simulink model "Time_example"  (R2015a)
settings: Solver=ode1  SolverMode=SingleTasking  StartTime=0.0  StopTime=Inf  FixedStep=0.0001  RelTol=1e-3
PostLoadFcn:
  | , if any(exist('dsrtsu_mdlpostloadfcn', 'file') == [2, 3, 6]), try dsrtsu_mdlpostloadfcn('Execute', bdroot); catch fprintf('Error in PostLoadFcn (dsrtsu_mdlpostloadfcn) for model "%s":\n %s\n', bdroot, lasterr); end, end,
libraries: rti1401lib_I_base x12, rtilib1401 x1
settings Model: RTICANMMDATA=struct('GeneralSetupData',struct('modelroot','E:\Support\RTI.2016.05.17.008','generalsettings',struct('filesettings',struct('destfolder',struct('Name','RTICANMM_FILES','Check',1),'buildfolder',struct('Name','.','Check',1),'AbsDestfolder',struct('Name','E:\Support\RTI.2016.05.17.008\RTICANMM_FILES'),'AbsBuildfolder',struct('Name','E:\Support\RTI.2016.05.17.008'))),'options',struct('addpaths',1,'rmpaths',1,'addtrcexclusion',logical(1),'cannavigator',struct('checkmonitoring',0),'show_usrtrc',0,'use_usrtrc',0),'advanced',struct('options',[1 1 1 1 1 1 1 1 1 1 1 1 1 1 1 1 1 1 1 1 1 1 1 1 1 1 1 1 1 1 1 1 1 1 1 1 1 1 1 1 1 1 1 1 1 1 1 1 1 1 1 1 1 1 1 1 1 1 1 1 1 1 1 1 1 1 1 1 1 1 1 1 1 1 1 1 1 1 1 1 1 1 1 1 1 1 1 1 1 1 1 1 1 1 1 1 1 1 1 1]),'MPSetup',{{}},'modelname','smd_1401_sl','block','smd_1401_sl'))  RTILINMMDATA=struct('GeneralSetupData',[])  DSRTSU_INTERNAL_RTI_VER=470  DSRTSU_INTERNAL_RTI_TYPE=rti1401  DSRTSU_INTERNAL_RTIFLEXRAYCONFIG=80  DSRTSU_INTERNAL_RTIFPGA=60  DSAPPLBUILDDATA=struct('workDir','E:\Support\RTI.2016.05.17.008','mpMainModel','smd_1401_sl','modelName','smd_1401_sl','isRTIMp',logical(0),'VerboseLevel',0,'modelHandle',3.000244140625,'mpMainHandle',3.000244140625,'buildDir','.\smd_1401_sl_rti1401','IsCodeGen',logical(1))  CovSFcnEnable=off  ExtModeTrigMode=oneshot  ExtModeArmWhenConnect=off  ExtModeAutoUpdateStatusClock=off  Creator=dSPACE GmbH  LastModifiedBy=Powertrain_software
settings DataIOCC: SignalLoggingSaveFormat=ModelDataLogs
settings OptimizationCC: BlockReduction=off  ConditionallyExecuteInputs=off  OptimizeBlockIOStorage=off  BufferReuse=off  GlobalBufferReuse=off  ExpressionFolding=off  ExpressionDepthLimit=2147483647  LocalBlockOutputs=off  InitFltsAndDblsToZero=on
settings DebuggingCC: SaveWithParameterizedLinksMsg=none  UnderspecifiedInitializationDetection=Classic  MergeDetectMultiDrivingBlocksExec=none  SignalResolutionControl=TryResolveAllWithWarning  SolverPrmCheckMsg=warning  MultiTaskDSMMsg=warning  MultiTaskCondExecSysMsg=none  MultiTaskRateTransMsg=warning  TasksWithSamePriorityMsg=none  FcnCallInpInsideContextMsg=UseLocalSettings  StateNameClashWarn=warning
settings HardwareCC: ProdLargestAtomicInteger=Integer  ProdLargestAtomicFloat=Float  ProdIntDivRoundTo=Zero  ProdEndianess=BigEndian  ProdHWDeviceType=Generic->Custom  TargetIntDivRoundTo=Zero  TargetEndianess=BigEndian  TargetHWDeviceType=Generic->Custom
settings RTWCC: SystemTargetFile=rti1401.tlc  MakeCommand=make_rti  TemplateMakefile=rti1401.tmf  Description=dSPACE DS1401 Hardware Platform  RTWVerbose=off
settings STFCustomTargetCC: TargetFcnLib=ansi_tfl_tmw.mat  GenerateSampleERTMain=off  ParMdlRefBuildCompliant=on  GeneratePreprocessorConditionals=Disable all  ERTCustomFileBanners=off  SupportNonInlinedSFcns=on  SupportVariableSizeSignals=off  MATLABClassNameForMDSCustomization=Simulink.SoftwareTarget.GRTCustomization  GRTInterface=on  SystemTargetFile=rti1401.tlc
settings GRTTargetCC: TargetFcnLib=ansi_tfl_tmw.mat  CompOptLevelCompliant=off  ConcurrentExecutionCompliant=off  CombineOutputUpdateFcns=off  MatFileLogging=off  CPPClassGenCompliant=off  GRTInterface=on  ExtModeMexFile=noextcomm

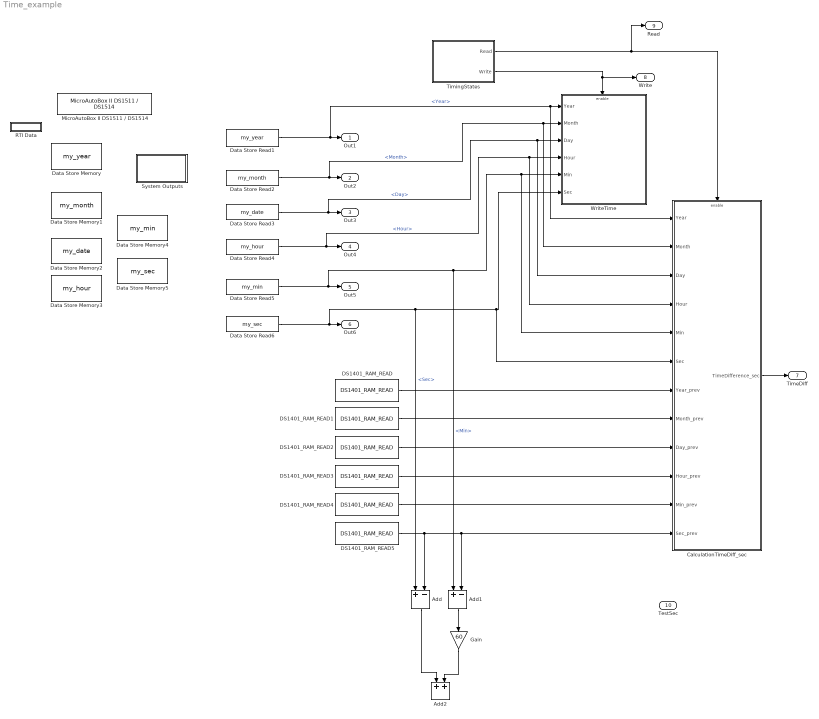
== system Time_example ==
  Add : Sum  Inputs=+-
  Add1 : Sum  Inputs=+-
  Add2 : Sum
  CalculationTimeDiff_sec : Subsystem  TreatAsAtomicUnit=on
  DS1401_RAM_READ : rti1401lib_I_base/DS1401_RAM_READ  DataType=Int8  Address=0  SampleTime=-1  Reserved1=[]  Reserved2=[]  Reserved3=[]  Reserved4=[]  DSProperties=struct('RTI',struct('Version',uint32(1),'BlockType',struct('isSLSource',uint8(1),'isSLSink',uint8(0),'isHWSource',uint8(0),'isHWSink',uint8(1),'isSetup',uint8(0),'isInline',uint8(1),'isNonInline',uint8(1),'isInterrupt',uint8(0),'isChannelwise',uint8(0)),'IOBoardType',{{'DS1401','BASE'}},'UnitType','RAM','Identifier','RAMREAD','DialogType','SL','BlockSet','NONE','SlaveProcessor','NONE'))  RTIBlockInterface=struct('OutputPortsActive',1,'BlockDisplay',{{['From\nnon-volatile RAM'],'center'}},'IconTransparency','off','InitLevel',1,'BlockName',struct('Token',{{'DS1401_RAM_READ'}}),'MaskDescription',['Provide read access from non-volatile Real-Time-Clock user RAM.'])  RTIBlockParameters=struct('DataType',{{1,'ON',[1 8]}},'Address',{{0,'ON','DataType',[0 1 2 3 4 5 6 7 8 9 10 11 12 13 14 15;0 1 2 3 4 5 6 7 8 9 10 11 12 13 14 15;0 0 2 2 4 4 6 6 8 8 10 10 12 12 14 14;0 0 2 2 4 4 6 6 8 8 10 10 12 12 14 14;0 0 0 0 4 4 4 4 8 8 8 8 12 12 12 12;0 0 0 0 4 4 4 4 8 8 8 8 12 12 12 12;0 0 0 0 4 4 4 4 8 8 8 8 12 12 12 12;0 0 0 0 0 0 0 0 8 8 8 8 8 8 8 8]}},'SampleTime',{{-1,'OFF',[]}})  RTISFcnParameters=struct('DataType','double','Address','double','SampleTime','double')  RTIBlockParaDefault=struct('DataType',8,'Address',0,'SampleTime',-1)
  DS1401_RAM_READ1 : rti1401lib_I_base/DS1401_RAM_READ  DataType=Int8  Address=1  SampleTime=-1  Reserved1=[]  Reserved2=[]  Reserved3=[]  Reserved4=[]  DSProperties=struct('RTI',struct('Version',uint32(1),'BlockType',struct('isSLSource',uint8(1),'isSLSink',uint8(0),'isHWSource',uint8(0),'isHWSink',uint8(1),'isSetup',uint8(0),'isInline',uint8(1),'isNonInline',uint8(1),'isInterrupt',uint8(0),'isChannelwise',uint8(0)),'IOBoardType',{{'DS1401','BASE'}},'UnitType','RAM','Identifier','RAMREAD','DialogType','SL','BlockSet','NONE','SlaveProcessor','NONE'))  RTIBlockInterface=struct('OutputPortsActive',1,'BlockDisplay',{{['From\nnon-volatile RAM'],'center'}},'IconTransparency','off','InitLevel',1,'BlockName',struct('Token',{{'DS1401_RAM_READ'}}),'MaskDescription',['Provide read access from non-volatile Real-Time-Clock user RAM.'])  RTIBlockParameters=struct('DataType',{{1,'ON',[1 8]}},'Address',{{1,'ON','DataType',[0 1 2 3 4 5 6 7 8 9 10 11 12 13 14 15;0 1 2 3 4 5 6 7 8 9 10 11 12 13 14 15;0 0 2 2 4 4 6 6 8 8 10 10 12 12 14 14;0 0 2 2 4 4 6 6 8 8 10 10 12 12 14 14;0 0 0 0 4 4 4 4 8 8 8 8 12 12 12 12;0 0 0 0 4 4 4 4 8 8 8 8 12 12 12 12;0 0 0 0 4 4 4 4 8 8 8 8 12 12 12 12;0 0 0 0 0 0 0 0 8 8 8 8 8 8 8 8]}},'SampleTime',{{-1,'OFF',[]}})  RTISFcnParameters=struct('DataType','double','Address','double','SampleTime','double')  RTIBlockParaDefault=struct('DataType',8,'Address',0,'SampleTime',-1)
  DS1401_RAM_READ2 : rti1401lib_I_base/DS1401_RAM_READ  DataType=Int8  Address=2  SampleTime=-1  Reserved1=[]  Reserved2=[]  Reserved3=[]  Reserved4=[]  DSProperties=struct('RTI',struct('Version',uint32(1),'BlockType',struct('isSLSource',uint8(1),'isSLSink',uint8(0),'isHWSource',uint8(0),'isHWSink',uint8(1),'isSetup',uint8(0),'isInline',uint8(1),'isNonInline',uint8(1),'isInterrupt',uint8(0),'isChannelwise',uint8(0)),'IOBoardType',{{'DS1401','BASE'}},'UnitType','RAM','Identifier','RAMREAD','DialogType','SL','BlockSet','NONE','SlaveProcessor','NONE'))  RTIBlockInterface=struct('OutputPortsActive',1,'BlockDisplay',{{['From\nnon-volatile RAM'],'center'}},'IconTransparency','off','InitLevel',1,'BlockName',struct('Token',{{'DS1401_RAM_READ'}}),'MaskDescription',['Provide read access from non-volatile Real-Time-Clock user RAM.'])  RTIBlockParameters=struct('DataType',{{1,'ON',[1 8]}},'Address',{{2,'ON','DataType',[0 1 2 3 4 5 6 7 8 9 10 11 12 13 14 15;0 1 2 3 4 5 6 7 8 9 10 11 12 13 14 15;0 0 2 2 4 4 6 6 8 8 10 10 12 12 14 14;0 0 2 2 4 4 6 6 8 8 10 10 12 12 14 14;0 0 0 0 4 4 4 4 8 8 8 8 12 12 12 12;0 0 0 0 4 4 4 4 8 8 8 8 12 12 12 12;0 0 0 0 4 4 4 4 8 8 8 8 12 12 12 12;0 0 0 0 0 0 0 0 8 8 8 8 8 8 8 8]}},'SampleTime',{{-1,'OFF',[]}})  RTISFcnParameters=struct('DataType','double','Address','double','SampleTime','double')  RTIBlockParaDefault=struct('DataType',8,'Address',0,'SampleTime',-1)
  DS1401_RAM_READ3 : rti1401lib_I_base/DS1401_RAM_READ  DataType=Int8  Address=3  SampleTime=-1  Reserved1=[]  Reserved2=[]  Reserved3=[]  Reserved4=[]  DSProperties=struct('RTI',struct('Version',uint32(1),'BlockType',struct('isSLSource',uint8(1),'isSLSink',uint8(0),'isHWSource',uint8(0),'isHWSink',uint8(1),'isSetup',uint8(0),'isInline',uint8(1),'isNonInline',uint8(1),'isInterrupt',uint8(0),'isChannelwise',uint8(0)),'IOBoardType',{{'DS1401','BASE'}},'UnitType','RAM','Identifier','RAMREAD','DialogType','SL','BlockSet','NONE','SlaveProcessor','NONE'))  RTIBlockInterface=struct('OutputPortsActive',1,'BlockDisplay',{{['From\nnon-volatile RAM'],'center'}},'IconTransparency','off','InitLevel',1,'BlockName',struct('Token',{{'DS1401_RAM_READ'}}),'MaskDescription',['Provide read access from non-volatile Real-Time-Clock user RAM.'])  RTIBlockParameters=struct('DataType',{{1,'ON',[1 8]}},'Address',{{3,'ON','DataType',[0 1 2 3 4 5 6 7 8 9 10 11 12 13 14 15;0 1 2 3 4 5 6 7 8 9 10 11 12 13 14 15;0 0 2 2 4 4 6 6 8 8 10 10 12 12 14 14;0 0 2 2 4 4 6 6 8 8 10 10 12 12 14 14;0 0 0 0 4 4 4 4 8 8 8 8 12 12 12 12;0 0 0 0 4 4 4 4 8 8 8 8 12 12 12 12;0 0 0 0 4 4 4 4 8 8 8 8 12 12 12 12;0 0 0 0 0 0 0 0 8 8 8 8 8 8 8 8]}},'SampleTime',{{-1,'OFF',[]}})  RTISFcnParameters=struct('DataType','double','Address','double','SampleTime','double')  RTIBlockParaDefault=struct('DataType',8,'Address',0,'SampleTime',-1)
  DS1401_RAM_READ4 : rti1401lib_I_base/DS1401_RAM_READ  DataType=Int8  Address=4  SampleTime=-1  Reserved1=[]  Reserved2=[]  Reserved3=[]  Reserved4=[]  DSProperties=struct('RTI',struct('Version',uint32(1),'BlockType',struct('isSLSource',uint8(1),'isSLSink',uint8(0),'isHWSource',uint8(0),'isHWSink',uint8(1),'isSetup',uint8(0),'isInline',uint8(1),'isNonInline',uint8(1),'isInterrupt',uint8(0),'isChannelwise',uint8(0)),'IOBoardType',{{'DS1401','BASE'}},'UnitType','RAM','Identifier','RAMREAD','DialogType','SL','BlockSet','NONE','SlaveProcessor','NONE'))  RTIBlockInterface=struct('OutputPortsActive',1,'BlockDisplay',{{['From\nnon-volatile RAM'],'center'}},'IconTransparency','off','InitLevel',1,'BlockName',struct('Token',{{'DS1401_RAM_READ'}}),'MaskDescription',['Provide read access from non-volatile Real-Time-Clock user RAM.'])  RTIBlockParameters=struct('DataType',{{1,'ON',[1 8]}},'Address',{{4,'ON','DataType',[0 1 2 3 4 5 6 7 8 9 10 11 12 13 14 15;0 1 2 3 4 5 6 7 8 9 10 11 12 13 14 15;0 0 2 2 4 4 6 6 8 8 10 10 12 12 14 14;0 0 2 2 4 4 6 6 8 8 10 10 12 12 14 14;0 0 0 0 4 4 4 4 8 8 8 8 12 12 12 12;0 0 0 0 4 4 4 4 8 8 8 8 12 12 12 12;0 0 0 0 4 4 4 4 8 8 8 8 12 12 12 12;0 0 0 0 0 0 0 0 8 8 8 8 8 8 8 8]}},'SampleTime',{{-1,'OFF',[]}})  RTISFcnParameters=struct('DataType','double','Address','double','SampleTime','double')  RTIBlockParaDefault=struct('DataType',8,'Address',0,'SampleTime',-1)
  DS1401_RAM_READ5 : rti1401lib_I_base/DS1401_RAM_READ  DataType=Int8  Address=5  SampleTime=-1  Reserved1=[]  Reserved2=[]  Reserved3=[]  Reserved4=[]  DSProperties=struct('RTI',struct('Version',uint32(1),'BlockType',struct('isSLSource',uint8(1),'isSLSink',uint8(0),'isHWSource',uint8(0),'isHWSink',uint8(1),'isSetup',uint8(0),'isInline',uint8(1),'isNonInline',uint8(1),'isInterrupt',uint8(0),'isChannelwise',uint8(0)),'IOBoardType',{{'DS1401','BASE'}},'UnitType','RAM','Identifier','RAMREAD','DialogType','SL','BlockSet','NONE','SlaveProcessor','NONE'))  RTIBlockInterface=struct('OutputPortsActive',1,'BlockDisplay',{{['From\nnon-volatile RAM'],'center'}},'IconTransparency','off','InitLevel',1,'BlockName',struct('Token',{{'DS1401_RAM_READ'}}),'MaskDescription',['Provide read access from non-volatile Real-Time-Clock user RAM.'])  RTIBlockParameters=struct('DataType',{{1,'ON',[1 8]}},'Address',{{5,'ON','DataType',[0 1 2 3 4 5 6 7 8 9 10 11 12 13 14 15;0 1 2 3 4 5 6 7 8 9 10 11 12 13 14 15;0 0 2 2 4 4 6 6 8 8 10 10 12 12 14 14;0 0 2 2 4 4 6 6 8 8 10 10 12 12 14 14;0 0 0 0 4 4 4 4 8 8 8 8 12 12 12 12;0 0 0 0 4 4 4 4 8 8 8 8 12 12 12 12;0 0 0 0 4 4 4 4 8 8 8 8 12 12 12 12;0 0 0 0 0 0 0 0 8 8 8 8 8 8 8 8]}},'SampleTime',{{-1,'OFF',[]}})  RTISFcnParameters=struct('DataType','double','Address','double','SampleTime','double')  RTIBlockParaDefault=struct('DataType',8,'Address',0,'SampleTime',-1)
  Data Store Memory : DataStoreMemory  DataStoreName=my_year  ReadBeforeWriteMsg=warning  WriteAfterWriteMsg=warning  WriteAfterReadMsg=warning
      settings: RTWStateStorageClass=ExportedGlobal
  Data Store Memory1 : DataStoreMemory  DataStoreName=my_month  ReadBeforeWriteMsg=warning  WriteAfterWriteMsg=warning  WriteAfterReadMsg=warning
      settings: RTWStateStorageClass=ExportedGlobal
  Data Store Memory2 : DataStoreMemory  DataStoreName=my_date  ReadBeforeWriteMsg=warning  WriteAfterWriteMsg=warning  WriteAfterReadMsg=warning
      settings: RTWStateStorageClass=ExportedGlobal
  Data Store Memory3 : DataStoreMemory  DataStoreName=my_hour  ReadBeforeWriteMsg=warning  WriteAfterWriteMsg=warning  WriteAfterReadMsg=warning
      settings: RTWStateStorageClass=ExportedGlobal
  Data Store Memory4 : DataStoreMemory  DataStoreName=my_min  ReadBeforeWriteMsg=warning  WriteAfterWriteMsg=warning  WriteAfterReadMsg=warning
      settings: RTWStateStorageClass=ExportedGlobal
  Data Store Memory5 : DataStoreMemory  DataStoreName=my_sec  ReadBeforeWriteMsg=warning  WriteAfterWriteMsg=warning  WriteAfterReadMsg=warning
      settings: RTWStateStorageClass=ExportedGlobal
  Data Store Read1 : DataStoreRead  DataStoreName=my_year
  Data Store Read2 : DataStoreRead  DataStoreName=my_month
  Data Store Read3 : DataStoreRead  DataStoreName=my_date
  Data Store Read4 : DataStoreRead  DataStoreName=my_hour
  Data Store Read5 : DataStoreRead  DataStoreName=my_min
  Data Store Read6 : DataStoreRead  DataStoreName=my_sec
  Gain : Gain  Gain=60
  MicroAutoBox II DS1511 / DS1514 : rtilib1401/MicroAutoBox II DS1511 // DS1514  SystemSampleTime=-1
  RTI Data : Subsystem  Tag=struct('RTIDataServer',struct('RTIDataServerVs','2','RTIModelDescription','struct(''main'',''Time_example'',''sub'','''',''isMp'',0)'))  LoadFcn="if exist('rtidc'), try,  rtidc('DataHostBlockClbLoad', gcbh); catch, disp(['Warning: ''LoadFcn'' for RTI Data block failed: ' lasterr]); end, end,"  mask(RTI_DATA_HOST){}
      mask help:
      | RTI Data Block.
      | This block is used by RTI to store internal model-dependent data.
      | Please keep this block on the root level of the model. Deleting this block will result in data loss.
      |
      | NEVER DELETE OR COPY THIS BLOCK!
      settings: CopyFcn="if exist('rtidc'), try,  rtidc('DataHostBlockClbCopy', gcbh); catch, disp(['Warning: ''CopyFcn'' for RTI Data block failed: ' lasterr]); end, end,"  DeleteFcn="if exist('rtidc'), try,  rtidc('DataHostBlockClbDelete', gcbh); catch, disp(['Warning: ''DeleteFcn'' for RTI Data block failed: ' lasterr]); end, end,"  ModelCloseFcn="if exist('rtidc'), try,  rtidc('DataHostBlockClbModelClose', gcbh); catch, disp(['Warning: ''ModelCloseFcn'' for RTI Data block failed: ' lasterr]); end, end,"  PreSaveFcn="if exist('rtidc'), try,  rtidc('DataHostBlockClbPreSave', gcbh); catch, disp(['Warning: ''PreSaveFcn'' for RTI Data block failed: ' lasterr]); end, end,"  PostSaveFcn="if exist('rtidc'), try,  rtidc('DataHostBlockClbPostSave', gcbh); catch, disp(['Warning: ''PostSaveFcn'' for RTI Data block failed: ' lasterr]); end, end,"  NameChangeFcn="if exist('rtidc'), try,  rtidc('DataHostBlockClbNameChange', gcbh); catch, disp(['Warning: ''NameChangeFcn'' for RTI Data block failed: ' lasterr]); end, end,"
      mask Help:
      | RTI Data Block.
      | This block is used by RTI to store internal model-dependent data.
      | Please keep this block on the root level of the model. Deleting this block will result in data loss.
      | 
      | NEVER DELETE OR COPY THIS BLOCK!
      mask Display:
      | text(0.5, 0.5, 'RTI Data', 'HorizontalAlignment', 'center');
      | plot([1 0]);
  System Outputs : Subsystem  mask(System Outputs){ShowInLibBrowser=0}
      mask prompts: ShowInLibBrowser "Simulink:masks:CustCodeMaskParam1_MP"
      settings: CopyFcn=cccopyfcn(gcb)  OpenFcn=ccopenfcn('System Outputs Function')
      mask Help: eval('feval(''rtwprivate'',''rtwhelpview'',''rtw_sys_outputs_block'')');
      mask Display: disp('System\nOutputs');
  TimingStates : Stateflow chart  TreatAsAtomicUnit=on
  WriteTime : Subsystem  TreatAsAtomicUnit=on
  Out1 : Outport
  Out2 : Outport  Port=2
  Out3 : Outport  Port=3
  Out4 : Outport  Port=4
  Out5 : Outport  Port=5
  Out6 : Outport  Port=6
  TimeDiff : Outport  Port=7
  Write : Outport  Port=8
  Read : Outport  Port=9
  TestSec : Outport  Port=10
  wires:
  TimingStates/1(Read) -> Read/1, CalculationTimeDiff_sec/Enable
  TimingStates/2(Write) -> Write/1, WriteTime/Enable
  Data Store Read1/1 -> CalculationTimeDiff_sec/1(Year), WriteTime/1(Year), Out1/1  "<Year>"
  Data Store Read5/1 -> Add1/1, CalculationTimeDiff_sec/5(Min), WriteTime/5(Min), Out5/1  "<Min>"
  Data Store Read4/1 -> CalculationTimeDiff_sec/4(Hour), WriteTime/4(Hour), Out4/1  "<Hour>"
  Data Store Read2/1 -> CalculationTimeDiff_sec/2(Month), WriteTime/2(Month), Out2/1  "<Month>"
  Data Store Read6/1 -> CalculationTimeDiff_sec/6(Sec), WriteTime/6(Sec), Add/1, Out6/1  "<Sec>"
  Data Store Read3/1 -> CalculationTimeDiff_sec/3(Day), WriteTime/3(Day), Out3/1  "<Day>"
  CalculationTimeDiff_sec/1(TimeDifference_sec) -> TimeDiff/1
  DS1401_RAM_READ5/1 -> CalculationTimeDiff_sec/12(Sec_prev), Add1/2, Add/2
  DS1401_RAM_READ4/1 -> CalculationTimeDiff_sec/11(Min_prev)
  DS1401_RAM_READ3/1 -> CalculationTimeDiff_sec/10(Hour_prev)
  DS1401_RAM_READ2/1 -> CalculationTimeDiff_sec/9(Day_prev)
  DS1401_RAM_READ1/1 -> CalculationTimeDiff_sec/8(Month_prev)
  DS1401_RAM_READ/1 -> CalculationTimeDiff_sec/7(Year_prev)
  Add1/1 -> Gain/1
  Add/1 -> Add2/1
  Gain/1 -> Add2/2

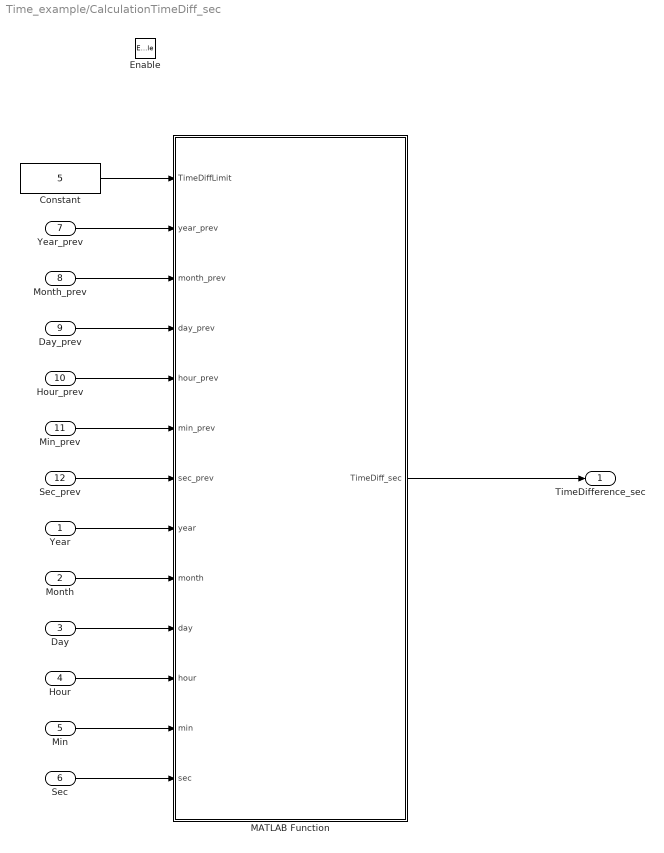
== system Time_example/CalculationTimeDiff_sec ==
  Year : Inport
  Month : Inport  Port=2
  Day : Inport  Port=3
  Hour : Inport  Port=4
  Min : Inport  Port=5
  Sec : Inport  Port=6
  Year_prev : Inport  Port=7
  Month_prev : Inport  Port=8
  Day_prev : Inport  Port=9
  Hour_prev : Inport  Port=10
  Min_prev : Inport  Port=11
  Sec_prev : Inport  Port=12
  Enable : EnablePort
  Constant : Constant  Value=5  OutDataTypeStr=int8
  MATLAB Function : MATLAB Function  TreatAsAtomicUnit=on
  TimeDifference_sec : Outport
  wires:
  MATLAB Function/1(TimeDiff_sec) -> TimeDifference_sec/1
  Constant/1 -> MATLAB Function/1(TimeDiffLimit)
  Sec_prev/1 -> MATLAB Function/7(sec_prev)
  Year/1 -> MATLAB Function/8(year)
  Month/1 -> MATLAB Function/9(month)
  Day/1 -> MATLAB Function/10(day)
  Hour/1 -> MATLAB Function/11(hour)
  Min/1 -> MATLAB Function/12(min)
  Sec/1 -> MATLAB Function/13(sec)
  Min_prev/1 -> MATLAB Function/6(min_prev)
  Day_prev/1 -> MATLAB Function/4(day_prev)
  Hour_prev/1 -> MATLAB Function/5(hour_prev)
  Month_prev/1 -> MATLAB Function/3(month_prev)
  Year_prev/1 -> MATLAB Function/2(year_prev)

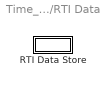
== system Time_example/RTI Data ==
  RTI Data Store : Subsystem  Tag="struct('private',struct('version',struct('dsVer',uint32(2),'dsVerCreation',uint32(2),'RTI',struct('ver','7.5p2','type','RTI1401')),'access',struct('type','Model','isPerm',1,'created',['19-May-2016 14:11:30'],'modified',['20-May-2016 18:16:36'],'location','')),'public',struct('main',struct('data',[]),'sub',struct('name',{{'Time_example'}},'data',{{struct('TH',struct('thTaskInfo',struct('taskType',{'TIMER','HWINT','TMRINT','SWINT','GLINT'},'tasksNumOf',{1,0,0,0,0},'srcIds',{{'TIMERA'},{},{},{},{}},'taskNames',{{['Timer Task 1']},{},{},{},{}})),'th_tc',struct('dataType','TASK','taskGroupId','','taskGroupList',{{}},'taskSchedulingPolicy','FCFS','taskType','TIMER','blkh',-1,'srcId','TIMERA','srcSgnName',['Timer A interrupt'],'srcCpuName','','taskName',['Timer Task 1  [0.0001] s'],'taskNameDisplayExt','','smplTime',0.0001,'smplTimeOffs',0,'hasFixedPriority',0,'priority',1,'hasFixedOvc',0,'ovcType',1,'ovcMax',1),'tc_th',struct('dataType','TASK','taskGroupId','','taskGroupList',{{}},'taskSchedulingPolicy','FCFS','taskType','TIMER','blkh',-1,'srcId','TIMERA','srcSgnName',['Timer A interrupt'],'srcCpuName','','taskName',['Timer Task 1  [0.0001] s'],'taskNameDisplayExt','','smplTime',0.0001,'smplTimeOffs',0,'hasFixedPriority',0,'priority',1,'hasFixedOvc',0,'ovcType',1,'ovcMax',1))}})))"  mask(RTI_DATA_STORE){}
      mask help:
      | RTI Data Store Block. This block is used by RTI to store internal model dependent data. Deleting this block will result in data loss.
      |
      | NEVER DELETE, COPY, OR MODIFY THIS BLOCK!
      mask Help:
      | RTI Data Store Block. This block is used by RTI to store internal model dependent data. Deleting this block will result in data loss.
      | 
      | NEVER DELETE, COPY, OR MODIFY THIS BLOCK!
      mask Display: text(0.5, 0.5, ' ', 'HorizontalAlignment', 'center');

== system Time_example/System Outputs ==

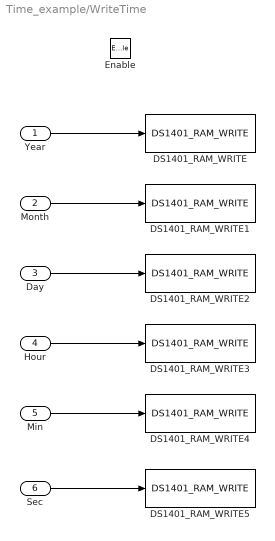
== system Time_example/WriteTime ==
  Year : Inport
  Month : Inport  Port=2
  Day : Inport  Port=3
  Hour : Inport  Port=4
  Min : Inport  Port=5
  Sec : Inport  Port=6
  Enable : EnablePort
  DS1401_RAM_WRITE : rti1401lib_I_base/DS1401_RAM_WRITE  DataType=Int8  Address=0  SampleTime=1  Reserved1=[]  Reserved2=[]  Reserved3=[]  Reserved4=[]  DSProperties=struct('RTI',struct('Version',uint32(1),'BlockType',struct('isSLSource',uint8(0),'isSLSink',uint8(1),'isHWSource',uint8(1),'isHWSink',uint8(1),'isSetup',uint8(0),'isInline',uint8(1),'isNonInline',uint8(1),'isInterrupt',uint8(0),'isChannelwise',uint8(0)),'IOBoardType',{{'DS1401','BASE'}},'UnitType','RAM','Identifier','RAMWRITE','DialogType','SL','BlockSet','NONE','SlaveProcessor','NONE'))  RTIBlockInterface=struct('InputPortsActive',1,'BlockDisplay',{{['To\nnon-volatile RAM'],'center'}},'IconTransparency','off','InitLevel',1,'BlockName',struct('Token',{{'DS1401_RAM_WRITE'}}),'MaskDescription',['Provide read access from non-volatile Real-Time-Clock user RAM.'])  RTIBlockParameters=struct('DataType',{{1,'ON',[1 8]}},'Address',{{0,'ON','DataType',[0 1 2 3 4 5 6 7 8 9 10 11 12 13 14 15;0 1 2 3 4 5 6 7 8 9 10 11 12 13 14 15;0 0 2 2 4 4 6 6 8 8 10 10 12 12 14 14;0 0 2 2 4 4 6 6 8 8 10 10 12 12 14 14;0 0 0 0 4 4 4 4 8 8 8 8 12 12 12 12;0 0 0 0 4 4 4 4 8 8 8 8 12 12 12 12;0 0 0 0 4 4 4 4 8 8 8 8 12 12 12 12;0 0 0 0 0 0 0 0 8 8 8 8 8 8 8 8]}},'SampleTime',{{1,'OFF',[]}})  RTISFcnParameters=struct('DataType','double','Address','double','SampleTime','double')  RTIBlockParaDefault=struct('DataType',8,'Address',0,'SampleTime',-1)
  DS1401_RAM_WRITE1 : rti1401lib_I_base/DS1401_RAM_WRITE  DataType=Int8  Address=1  SampleTime=1  Reserved1=[]  Reserved2=[]  Reserved3=[]  Reserved4=[]  DSProperties=struct('RTI',struct('Version',uint32(1),'BlockType',struct('isSLSource',uint8(0),'isSLSink',uint8(1),'isHWSource',uint8(1),'isHWSink',uint8(1),'isSetup',uint8(0),'isInline',uint8(1),'isNonInline',uint8(1),'isInterrupt',uint8(0),'isChannelwise',uint8(0)),'IOBoardType',{{'DS1401','BASE'}},'UnitType','RAM','Identifier','RAMWRITE','DialogType','SL','BlockSet','NONE','SlaveProcessor','NONE'))  RTIBlockInterface=struct('InputPortsActive',1,'BlockDisplay',{{['To\nnon-volatile RAM'],'center'}},'IconTransparency','off','InitLevel',1,'BlockName',struct('Token',{{'DS1401_RAM_WRITE'}}),'MaskDescription',['Provide read access from non-volatile Real-Time-Clock user RAM.'])  RTIBlockParameters=struct('DataType',{{1,'ON',[1 8]}},'Address',{{1,'ON','DataType',[0 1 2 3 4 5 6 7 8 9 10 11 12 13 14 15;0 1 2 3 4 5 6 7 8 9 10 11 12 13 14 15;0 0 2 2 4 4 6 6 8 8 10 10 12 12 14 14;0 0 2 2 4 4 6 6 8 8 10 10 12 12 14 14;0 0 0 0 4 4 4 4 8 8 8 8 12 12 12 12;0 0 0 0 4 4 4 4 8 8 8 8 12 12 12 12;0 0 0 0 4 4 4 4 8 8 8 8 12 12 12 12;0 0 0 0 0 0 0 0 8 8 8 8 8 8 8 8]}},'SampleTime',{{1,'OFF',[]}})  RTISFcnParameters=struct('DataType','double','Address','double','SampleTime','double')  RTIBlockParaDefault=struct('DataType',8,'Address',0,'SampleTime',-1)
  DS1401_RAM_WRITE2 : rti1401lib_I_base/DS1401_RAM_WRITE  DataType=Int8  Address=2  SampleTime=1  Reserved1=[]  Reserved2=[]  Reserved3=[]  Reserved4=[]  DSProperties=struct('RTI',struct('Version',uint32(1),'BlockType',struct('isSLSource',uint8(0),'isSLSink',uint8(1),'isHWSource',uint8(1),'isHWSink',uint8(1),'isSetup',uint8(0),'isInline',uint8(1),'isNonInline',uint8(1),'isInterrupt',uint8(0),'isChannelwise',uint8(0)),'IOBoardType',{{'DS1401','BASE'}},'UnitType','RAM','Identifier','RAMWRITE','DialogType','SL','BlockSet','NONE','SlaveProcessor','NONE'))  RTIBlockInterface=struct('InputPortsActive',1,'BlockDisplay',{{['To\nnon-volatile RAM'],'center'}},'IconTransparency','off','InitLevel',1,'BlockName',struct('Token',{{'DS1401_RAM_WRITE'}}),'MaskDescription',['Provide read access from non-volatile Real-Time-Clock user RAM.'])  RTIBlockParameters=struct('DataType',{{1,'ON',[1 8]}},'Address',{{2,'ON','DataType',[0 1 2 3 4 5 6 7 8 9 10 11 12 13 14 15;0 1 2 3 4 5 6 7 8 9 10 11 12 13 14 15;0 0 2 2 4 4 6 6 8 8 10 10 12 12 14 14;0 0 2 2 4 4 6 6 8 8 10 10 12 12 14 14;0 0 0 0 4 4 4 4 8 8 8 8 12 12 12 12;0 0 0 0 4 4 4 4 8 8 8 8 12 12 12 12;0 0 0 0 4 4 4 4 8 8 8 8 12 12 12 12;0 0 0 0 0 0 0 0 8 8 8 8 8 8 8 8]}},'SampleTime',{{1,'OFF',[]}})  RTISFcnParameters=struct('DataType','double','Address','double','SampleTime','double')  RTIBlockParaDefault=struct('DataType',8,'Address',0,'SampleTime',-1)
  DS1401_RAM_WRITE3 : rti1401lib_I_base/DS1401_RAM_WRITE  DataType=Int8  Address=3  SampleTime=1  Reserved1=[]  Reserved2=[]  Reserved3=[]  Reserved4=[]  DSProperties=struct('RTI',struct('Version',uint32(1),'BlockType',struct('isSLSource',uint8(0),'isSLSink',uint8(1),'isHWSource',uint8(1),'isHWSink',uint8(1),'isSetup',uint8(0),'isInline',uint8(1),'isNonInline',uint8(1),'isInterrupt',uint8(0),'isChannelwise',uint8(0)),'IOBoardType',{{'DS1401','BASE'}},'UnitType','RAM','Identifier','RAMWRITE','DialogType','SL','BlockSet','NONE','SlaveProcessor','NONE'))  RTIBlockInterface=struct('InputPortsActive',1,'BlockDisplay',{{['To\nnon-volatile RAM'],'center'}},'IconTransparency','off','InitLevel',1,'BlockName',struct('Token',{{'DS1401_RAM_WRITE'}}),'MaskDescription',['Provide read access from non-volatile Real-Time-Clock user RAM.'])  RTIBlockParameters=struct('DataType',{{1,'ON',[1 8]}},'Address',{{3,'ON','DataType',[0 1 2 3 4 5 6 7 8 9 10 11 12 13 14 15;0 1 2 3 4 5 6 7 8 9 10 11 12 13 14 15;0 0 2 2 4 4 6 6 8 8 10 10 12 12 14 14;0 0 2 2 4 4 6 6 8 8 10 10 12 12 14 14;0 0 0 0 4 4 4 4 8 8 8 8 12 12 12 12;0 0 0 0 4 4 4 4 8 8 8 8 12 12 12 12;0 0 0 0 4 4 4 4 8 8 8 8 12 12 12 12;0 0 0 0 0 0 0 0 8 8 8 8 8 8 8 8]}},'SampleTime',{{1,'OFF',[]}})  RTISFcnParameters=struct('DataType','double','Address','double','SampleTime','double')  RTIBlockParaDefault=struct('DataType',8,'Address',0,'SampleTime',-1)
  DS1401_RAM_WRITE4 : rti1401lib_I_base/DS1401_RAM_WRITE  DataType=Int8  Address=4  SampleTime=1  Reserved1=[]  Reserved2=[]  Reserved3=[]  Reserved4=[]  DSProperties=struct('RTI',struct('Version',uint32(1),'BlockType',struct('isSLSource',uint8(0),'isSLSink',uint8(1),'isHWSource',uint8(1),'isHWSink',uint8(1),'isSetup',uint8(0),'isInline',uint8(1),'isNonInline',uint8(1),'isInterrupt',uint8(0),'isChannelwise',uint8(0)),'IOBoardType',{{'DS1401','BASE'}},'UnitType','RAM','Identifier','RAMWRITE','DialogType','SL','BlockSet','NONE','SlaveProcessor','NONE'))  RTIBlockInterface=struct('InputPortsActive',1,'BlockDisplay',{{['To\nnon-volatile RAM'],'center'}},'IconTransparency','off','InitLevel',1,'BlockName',struct('Token',{{'DS1401_RAM_WRITE'}}),'MaskDescription',['Provide read access from non-volatile Real-Time-Clock user RAM.'])  RTIBlockParameters=struct('DataType',{{1,'ON',[1 8]}},'Address',{{4,'ON','DataType',[0 1 2 3 4 5 6 7 8 9 10 11 12 13 14 15;0 1 2 3 4 5 6 7 8 9 10 11 12 13 14 15;0 0 2 2 4 4 6 6 8 8 10 10 12 12 14 14;0 0 2 2 4 4 6 6 8 8 10 10 12 12 14 14;0 0 0 0 4 4 4 4 8 8 8 8 12 12 12 12;0 0 0 0 4 4 4 4 8 8 8 8 12 12 12 12;0 0 0 0 4 4 4 4 8 8 8 8 12 12 12 12;0 0 0 0 0 0 0 0 8 8 8 8 8 8 8 8]}},'SampleTime',{{1,'OFF',[]}})  RTISFcnParameters=struct('DataType','double','Address','double','SampleTime','double')  RTIBlockParaDefault=struct('DataType',8,'Address',0,'SampleTime',-1)
  DS1401_RAM_WRITE5 : rti1401lib_I_base/DS1401_RAM_WRITE  DataType=Int8  Address=5  SampleTime=1  Reserved1=[]  Reserved2=[]  Reserved3=[]  Reserved4=[]  DSProperties=struct('RTI',struct('Version',uint32(1),'BlockType',struct('isSLSource',uint8(0),'isSLSink',uint8(1),'isHWSource',uint8(1),'isHWSink',uint8(1),'isSetup',uint8(0),'isInline',uint8(1),'isNonInline',uint8(1),'isInterrupt',uint8(0),'isChannelwise',uint8(0)),'IOBoardType',{{'DS1401','BASE'}},'UnitType','RAM','Identifier','RAMWRITE','DialogType','SL','BlockSet','NONE','SlaveProcessor','NONE'))  RTIBlockInterface=struct('InputPortsActive',1,'BlockDisplay',{{['To\nnon-volatile RAM'],'center'}},'IconTransparency','off','InitLevel',1,'BlockName',struct('Token',{{'DS1401_RAM_WRITE'}}),'MaskDescription',['Provide read access from non-volatile Real-Time-Clock user RAM.'])  RTIBlockParameters=struct('DataType',{{1,'ON',[1 8]}},'Address',{{5,'ON','DataType',[0 1 2 3 4 5 6 7 8 9 10 11 12 13 14 15;0 1 2 3 4 5 6 7 8 9 10 11 12 13 14 15;0 0 2 2 4 4 6 6 8 8 10 10 12 12 14 14;0 0 2 2 4 4 6 6 8 8 10 10 12 12 14 14;0 0 0 0 4 4 4 4 8 8 8 8 12 12 12 12;0 0 0 0 4 4 4 4 8 8 8 8 12 12 12 12;0 0 0 0 4 4 4 4 8 8 8 8 12 12 12 12;0 0 0 0 0 0 0 0 8 8 8 8 8 8 8 8]}},'SampleTime',{{1,'OFF',[]}})  RTISFcnParameters=struct('DataType','double','Address','double','SampleTime','double')  RTIBlockParaDefault=struct('DataType',8,'Address',0,'SampleTime',-1)
  wires:
  Year/1 -> DS1401_RAM_WRITE/1
  Month/1 -> DS1401_RAM_WRITE1/1
  Day/1 -> DS1401_RAM_WRITE2/1
  Hour/1 -> DS1401_RAM_WRITE3/1
  Min/1 -> DS1401_RAM_WRITE4/1
  Sec/1 -> DS1401_RAM_WRITE5/1

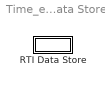
== system Time_example/RTI Data/RTI Data Store ==
  RTI Data Store : Subsystem  mask(RTI_DATA_STORE){}
      mask help:
      | RTI Data Store Block. This block is used by RTI to store internal model dependent data. Deleting this block will result in data loss.
      |
      | NEVER DELETE, COPY, OR MODIFY THIS BLOCK!
      mask Help:
      | RTI Data Store Block. This block is used by RTI to store internal model dependent data. Deleting this block will result in data loss.
      | 
      | NEVER DELETE, COPY, OR MODIFY THIS BLOCK!
      mask Display: text(0.5, 0.5, ' ', 'HorizontalAlignment', 'center');

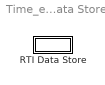
== system Time_example/RTI Data/RTI Data Store/RTI Data Store ==
  RTI Data Store : Subsystem  mask(RTI_DATA_STORE){}
      mask help:
      | RTI Data Store Block. This block is used by RTI to store internal model dependent data. Deleting this block will result in data loss.
      |
      | NEVER DELETE, COPY, OR MODIFY THIS BLOCK!
      mask Help:
      | RTI Data Store Block. This block is used by RTI to store internal model dependent data. Deleting this block will result in data loss.
      | 
      | NEVER DELETE, COPY, OR MODIFY THIS BLOCK!
      mask Display: text(0.5, 0.5, ' ', 'HorizontalAlignment', 'center');

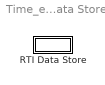
== system Time_example/RTI Data/RTI Data Store/RTI Data Store/RTI Data Store ==
  RTI Data Store : Subsystem  mask(RTI_DATA_STORE){}
      mask help:
      | RTI Data Store Block. This block is used by RTI to store internal model dependent data. Deleting this block will result in data loss.
      |
      | NEVER DELETE, COPY, OR MODIFY THIS BLOCK!
      mask Help:
      | RTI Data Store Block. This block is used by RTI to store internal model dependent data. Deleting this block will result in data loss.
      | 
      | NEVER DELETE, COPY, OR MODIFY THIS BLOCK!
      mask Display: text(0.5, 0.5, ' ', 'HorizontalAlignment', 'center');

== system Time_example/RTI Data/RTI Data Store/RTI Data Store/RTI Data Store/RTI Data Store ==

== stateflow chart Time_example/TimingStates ==
  state Initial
    during:
    Read = true;
    Write = false;
  state During
    during:
    Read = false;
    Write = true;
  (default) -> Initial
  Initial -> During : after (30,sec)
  data: Read output; Write output

== matlab function Time_example/CalculationTimeDiff_sec/MATLAB Function ==
  data: TimeDiffLimit input; year_prev input; TimeDiff_sec output; month_prev input; day_prev input; hour_prev input; min_prev input; sec_prev input; year input; month input; day input; hour input; min input; sec input
function TimeDiff_sec = TimeDifferenceCalculator(TimeDiffLimit,year_prev,month_prev,day_prev,hour_prev,min_prev,sec_prev,year,month,day,hour,min,sec)

% Total seconds measurement
if year_prev == year
%     t_prev = month_prev*3600*24*30 + day_prev*3600*24 + hour_prev*3600 + min_prev*60 + sec_prev;   
%     t = month*3600*24*30 + day*3600*24 + hour*3600 + min*60 + sec;
%     TimeDiff_sec = double(t - t_prev);
        t_prev = min_prev*60 + sec_prev;
        t = min*60 + sec;
        TimeDiff_sec = (t - t_prev);
else
    TimeDiff_sec = 2*TimeDiffLimit;
end
